simulink model "hdlFrame_AudioHighPassFilter_MLFB"  (R2022b)
settings: Solver=VariableStepAuto  StartTime=0.0  StopTime=0  RelTol=1e-3
InitFcn:
  | load chirp.mat;
undefined symbols (not defined in the file or in its folder): Fs, y
settings Model: Creator=quangha  LastModifiedBy=acuadros
settings SolverCC: MaxZcPerStep=1
settings OptimizationCC: BlockReduction=off  ConditionallyExecuteInputs=off  DefaultParameterBehavior=Inlined
settings DebuggingCC: AlgebraicLoopMsg=error
settings HardwareCC: ProdBitPerPointer=32  ProdBitPerSizeT=32  ProdBitPerPtrDiffT=32  ProdLargestAtomicFloat=None  ProdIntDivRoundTo=Undefined  ProdEndianess=Unspecified  ProdWordSize=32  ProdHWDeviceType=ASIC/FPGA->ASIC/FPGA  TargetBitPerPointer=64  TargetBitPerSizeT=64  TargetBitPerPtrDiffT=64  TargetLongLongMode=on  TargetIntDivRoundTo=Zero  TargetEndianess=LittleEndian  TargetWordSize=64  TargetHWDeviceType=Custom Processor->MATLAB Host Computer  ProdEqTarget=off
settings RTWCC: PlatformDefinition=Embedded Code

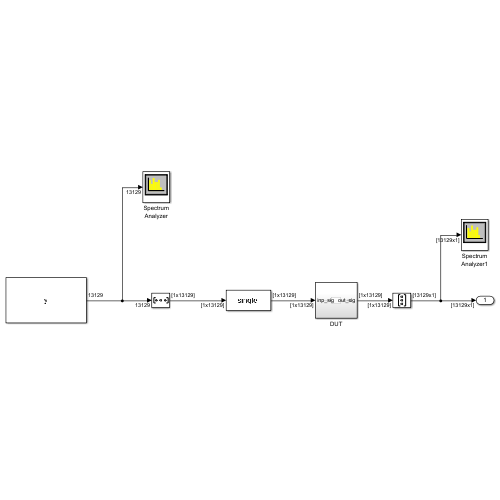
[thumbnail: Simulink's stored preview of the top-level diagram]
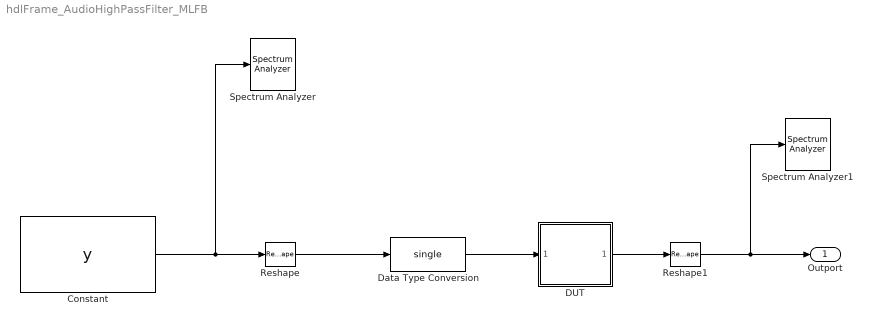
== system hdlFrame_AudioHighPassFilter_MLFB ==
  Constant : Constant  Value=y  SampleTime=1/Fs
  DUT : Subsystem
  Data Type Conversion : DataTypeConversion  OutDataTypeStr=single  SaturateOnIntegerOverflow=off  RndMeth=Floor
  Reshape : Reshape  OutputDimensionality=Row vector (2-D)
  Reshape1 : Reshape  OutputDimensionality=Column vector (2-D)
  Spectrum Analyzer : SpectrumAnalyzer
  Spectrum Analyzer1 : SpectrumAnalyzer
  Outport : Outport
  wires:
  DUT/1(out_sig) -> Reshape1/1
  Data Type Conversion/1 -> DUT/1(inp_sig)
  Constant/1 -> Reshape/1, Spectrum Analyzer/1
  Reshape/1 -> Data Type Conversion/1
  Reshape1/1 -> Spectrum Analyzer1/1, Outport/1

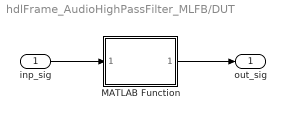
== system hdlFrame_AudioHighPassFilter_MLFB/DUT ==
  inp_sig : Inport
  MATLAB Function : MATLAB Function  TreatAsAtomicUnit=on
  out_sig : Outport
  wires:
  inp_sig/1 -> MATLAB Function/1(inp_sig)
  MATLAB Function/1(out_sig) -> out_sig/1

== matlab function hdlFrame_AudioHighPassFilter_MLFB/DUT/MATLAB Function ==
  data: inp_sig input; out_sig output
function out_sig = highpass_filter(inp_sig)

out_sig = hdl.npufun(@highpass_kernel, [1; 35], inp_sig);

end

function out = highpass_kernel(in)
hN = single(fir1(34,0.32,'high',chebwin(35,30)));
out = sum(in(:).*hN(:), 'native');
end
